simulink model "dev_RigTest"  (R2020b)
settings: Solver=VariableStepAuto  StartTime=0.0  StopTime=800  RelTol=1e-3
model workspace (MAT data in the model file):
  G_sup_tsp = Simulink.Signal
  G_sup_tsp.DataType = 'double'
  G_sup_tsp.Dimensions = -1
  G_sup_tsp.DimensionsMode = 'auto'
  G_sup_tsp.Complexity = 'real'
  G_sup_tsp.SampleTime = -1
  G_sup_tsp.SamplingMode = 'auto'
  G_sup_tsp.InitialValue = '175'
libraries: IMT_Library x3, simulink_extras x2, slpidlib x1
settings Model: Creator=Mr_Li  LastModifiedBy=Mr_Li

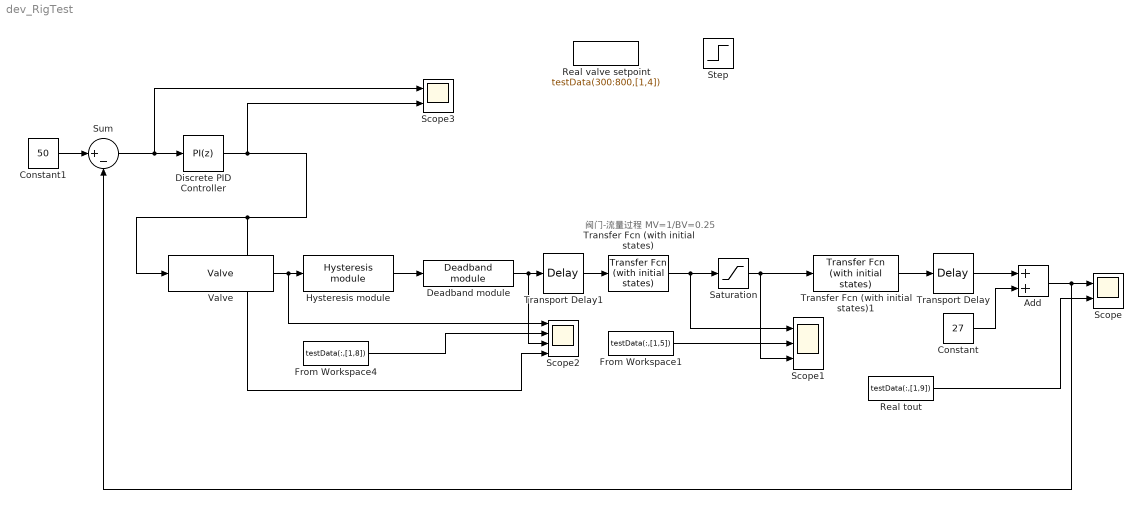
== system dev_RigTest ==
  note: 阀门-流量过程
      | MV=1/BV=0.25
  Add : Sum
  Constant : Constant  Value=27
  Constant1 : Constant  Value=50
  Deadband module : IMT_Library/Deadband module  upper=22.5  lower=6.5
      settings: SourceProductName=Imitation
  Discrete PID Controller : slpidlib/PID Controller  Controller=PI  Form=Parallel  TimeDomain=Discrete-time  UseExternalTs=off  SampleTime=1  IntegratorMethod=Forward Euler  FilterMethod=Forward Euler  ControllerParametersSource=internal  P=0.75  I=0.01  D=0  UseFilter=on  N=100  TunerSelectOption=Frequency Response Based  InitialConditionSource=internal  InitialConditionForIntegrator=0  InitialConditionForFilter=0  DifferentiatorICPrevScaledInput=0  ExternalReset=none  TrackingMode=off  Kt=1  LimitOutput=off  SatLimitsSource=internal  UpperSaturationLimit=inf  LowerSaturationLimit=-inf  LinearizeAsGain=off  AntiWindupMode=none  Kb=1  POutMin=[]  POutMax=[]  IOutMin=[]  IOutMax=[]  DOutMin=[]  DOutMax=[]  NOutMin=[]  NOutMax=[]  SumOutMin=[]  SumOutMax=[]  SaturationOutMin=[]  SaturationOutMax=[]  PParamMin=[]  PParamMax=[]  IParamMin=[]  IParamMax=[]  DParamMin=[]  DParamMax=[]  NParamMin=[]  NParamMax=[]  KbParamMin=[]  KbParamMax=[]  KtParamMin=[]  KtParamMax=[]  KbOutMin=[]  KbOutMax=[]  KtOutMin=[]  KtOutMax=[]  IntegratorOutMin=[]  IntegratorOutMax=[]  FilterOutMin=[]  FilterOutMax=[]  SumI1OutMin=[]  SumI1OutMax=[]  SumI2OutMin=[]  SumI2OutMax=[]  SumI3OutMin=[]  SumI3OutMax=[]  SumI4OutMin=[]  SumI4OutMax=[]  SumDOutMin=[]  SumDOutMax=[]  DifferentiatorOutMin=[]  DifferentiatorOutMax=[]  FilterDiffOutCoefMin=[]  FilterDiffOutCoefMax=[]  ReciprocalOutMin=[]  ReciprocalOutMax=[]  SumDenOutMin=[]  SumDenOutMax=[]  SumNumOutMin=[]  SumNumOutMax=[]  DivideOutMin=[]  DivideOutMax=[]  UdiffTsProdOutMin=[]  UdiffTsProdOutMax=[]  NTsProdOutMin=[]  NTsProdOutMax=[]  UintegralTsProdOutMin=[]  UintegralTsProdOutMax=[]  UngainTsProdOutMin=[]  UngainTsProdOutMax=[]  IntegratorContinuousStateAttributes=''  IntegratorStateMustResolveToSignalObject=off  IntegratorRTWStateStorageClass=Auto  FilterContinuousStateAttributes=''  FilterStateMustResolveToSignalObject=off  FilterRTWStateStorageClass=Auto  ParallelPVariant=InternalParameters  IdealPVariant=Disabled  IVariant=InternalParameters  DVariant=Disabled  IntegratorVariant=Discrete  SatVariant=Disabled  AWVariant=Passthrough  PCopyVariant=Disabled  TRVariant=Disabled  FdbkBlocksVariant=Forward  IdealPFdbkVariant=Disabled  SatFdbkVariant=Disabled  DerivativeFilterVariant=Disabled  NVariant=Disabled  NCopyVariant=Disabled_SignalSpec  FilterICVariant=Disabled  IntegratorICVariant=InternalICs  ExternalResetVariant=Disabled  TRSumVariant=Passthrough  SumFdbkVariant=Disabled  SumVariant=Sum_PI  TsampFilterVariant=InternalTs  TsampNgainVariant=Passthrough  TsampIntegralVariant=Passthrough  ExternalSaturationOutDataTypeStr=Inherit: Same as second input
  From Workspace1 : FromWorkspace  VariableName=testData(:,[1,5])
  From Workspace4 : FromWorkspace  VariableName=testData(:,[1,8])  SampleTime=1
  Hysteresis module : IMT_Library/Hysteresis module  hysteresisSize=4.5
      settings: SourceProductName=Imitation
  Real tout : FromWorkspace  VariableName=testData(:,[1,9])
  Real valve setpoint : FromWorkspace  VariableName=testData(300:800,[1,4])  SampleTime=1
  Saturation : Saturate  UpperLimit=0.25  LowerLimit=0
  Scope : Scope  NumInputPorts=2
  Scope1 : Scope  NumInputPorts=3
  Scope2 : Scope  NumInputPorts=4
  Scope3 : Scope  NumInputPorts=2
  Step : Step  Time=18  After=0.31  SampleTime=0
  Sum : Sum  Inputs=|+-
  Transfer Fcn (with initial states) : simulink_extras/Additional Linear/Transfer Fcn (with initial states)  N=[0.032]  D=[3.6 1]  X0=0
  Transfer Fcn (with initial states)1 : simulink_extras/Additional Linear/Transfer Fcn (with initial states)  N=[105]  D=[380 40 1]  X0=0
  Transport Delay : TransportDelay  DelayTime=0
  Transport Delay1 : TransportDelay  DelayTime=3
  Valve : IMT_Library/Valve  upper=101  lower=1.2  movementThreshold=1
      settings: SourceProductName=Imitation
  wires:
  Transport Delay1/1 -> Transfer Fcn (with initial states)/1
  Deadband module/1 -> Scope2/3, Transport Delay1/1
  Hysteresis module/1 -> Deadband module/1
  Valve/1 -> Scope2/1, Hysteresis module/1
  From Workspace1/1 -> Scope1/2
  Transfer Fcn (with initial states)1/1 -> Transport Delay/1
  Transport Delay/1 -> Add/1
  Constant/1 -> Add/2
  Add/1 -> Scope/1, Sum/2
  Saturation/1 -> Scope1/3, Transfer Fcn (with initial states)1/1
  From Workspace4/1 -> Scope2/2
  Sum/1 -> Scope3/1, Discrete PID Controller/1
  Discrete PID Controller/1 -> Scope3/2, Scope2/4, Valve/1
  Constant1/1 -> Sum/1
  Real tout/1 -> Scope/2
  Transfer Fcn (with initial states)/1 -> Scope1/1, Saturation/1
